simulink model "D2"  (R2019b)
settings: Solver=ode8  StartTime=0.0  StopTime=2  FixedStep=0.001000  RelTol=1e-3
settings Model: Creator=nahkusaidy  LastModifiedBy=nahkusaidy

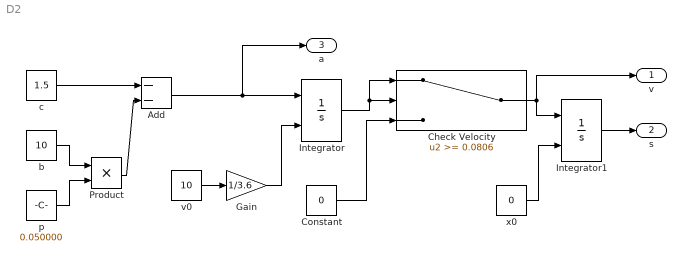
== system D2 ==
  Add : Sum  Inputs=--
  Check Velocity : Switch  Threshold=0.0806
  Constant : Constant  Value=0
  Gain : Gain  Gain=1/3.6
  Integrator : Integrator  InitialConditionSource=external
  Integrator1 : Integrator  InitialConditionSource=external
  Product : Product
  b : Constant  Value=10
  c : Constant  Value=1.5
  p : Constant  Value=0.050000
  v0 : Constant  Value=10
  x0 : Constant  Value=0
  v : Outport
  "s " : Outport  Port=2
  a : Outport  Port=3
  wires:
  c/1 -> Add/1
  b/1 -> Product/1
  p/1 -> Product/2
  Product/1 -> Add/2
  Integrator/1 -> Check Velocity/1, Check Velocity/2
  Integrator1/1 -> "s "/1
  x0/1 -> Integrator1/2
  v0/1 -> Gain/1
  Gain/1 -> Integrator/2
  Constant/1 -> Check Velocity/3
  Check Velocity/1 -> Integrator1/1, v/1
  Add/1 -> a/1, Integrator/1
